simulink library "TTLibrary"  (R2015a)
settings: Solver=ode45  StartTime=0.0  StopTime=10.0  RelTol=1e-3
undefined symbols (not defined in the file): addNoise, aHeat, Area, b, cp, inputOpt, kl, Kv, L1i, p, sampleTime, T1i, tPause, uT1
settings Model: CovSFcnEnable=off  Creator=blindner  LastModifiedBy=blindner
settings DebuggingCC: SolverPrmCheckMsg=warning

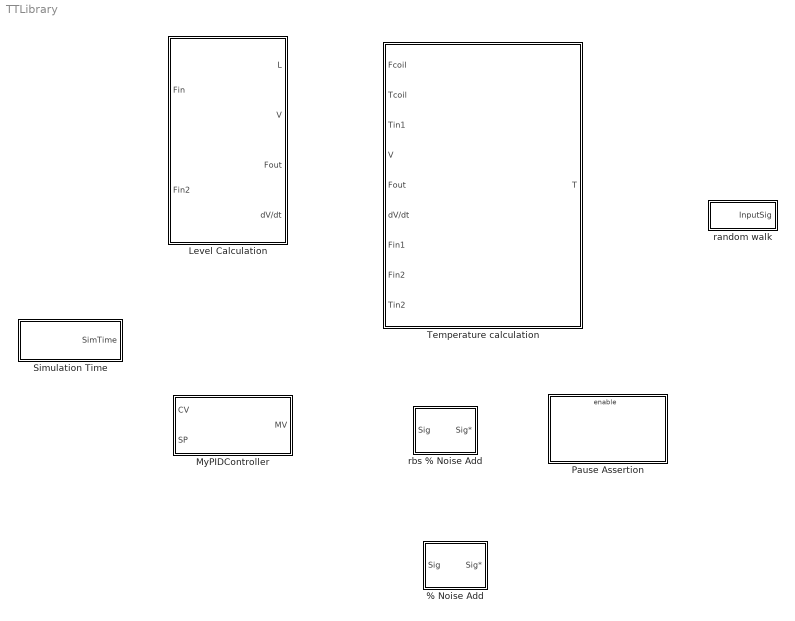
== system TTLibrary ==
  % Noise Add : Subsystem  mask{perc=5, seed=randi(100000), addNoiseMult=addNoise, Ts=sampleTime, noiseAmp=0}
      mask prompts: perc "Percentage Noise Added"; addNoiseMult "Add Noise: 0 or 1"; Ts "Sample Time"; noiseAmp "Amplitude of Noise added"
      mask Display: fprintf('AddNoise')
  Level Calculation : Subsystem  mask{kl=kl, Area=Area, Li=L1i, numIn=2}
      mask prompts: kl "Proportionality Constant"; Area "Cross-sectional Area"; Li "Initial Level"; numIn "Number of inports"
      mask init:
      | block = find_system(gcb,...
      |     'LookUnderMasks','on',...
      |     'FollowLinks','on','Name','Fin2');
      | 
      | switch numIn
      |     case '1'
      |         if ~isempty(block)
      |             delete_line(gcb,'Fin2/1','Sum/3');
      |             delete_block(block);
      |             set_param([gcb,'/Sum'],'Inputs','|+-')
      |         end
      |     case '2'
      |         if isempty(block)
      |             add_block('built-in/Inport',[gcb,'/Fin2'], 'Position',[155 190 175 210]);
      |            
      |             set_param([gcb,'/Sum'],'Inputs','+-+')
      |             add_line(gcb,'Fin2/1','Sum/3','autorouting','on');
      |             
      |         end
      | end % switch
      mask TypeOptions numIn: 1 | 2
  MyPIDController : Subsystem  mask{Kc=0, TI=0, Td=0, kv=0}
      mask prompts: Kc "Controller Gain"; TI "Integral Time"; Td "Derivative Time"; kv "Valve Constant"
      mask DialogControl DescTextVar Prompt: MV(s)=Kc*(1+1/TIs+Tds)*E(s)
  Pause Assertion : Subsystem
  Simulation Time : Subsystem  Variant=on  OverrideUsingVariant=Variant
  Temperature calculation : Subsystem  mask{Ti=T1i, p=p, cp=cp, b=b, aHeat=aHeat, numIn=2}
      mask prompts: Ti "Initial Temperature"; p "Density"; cp "Heat Capacity"; b "b: Heat transfer coeff costant"; aHeat "aHeat: Heat transfer coeff constant"; numIn "Number of Inports"
      mask init:
      | block = find_system(gcb,...
      |     'LookUnderMasks','on',...
      |     'FollowLinks','on','Name','Fin2');
      | 
      | switch numIn
      |     case '1'
      |         if ~isempty(block)
      |             delete_line(gcb,'Fin2/1','NewProduct/1');
      |             delete_line(gcb,'Tin2/1','NewProduct/2');
      |             delete_line(gcb,'NewProduct/1','Sum4/4');
      |             delete_block(block);
      |             delete_block([gcb,'/Tin2']);
      |             delete_block([gcb,'/NewProduct']);
      |             set_param([gcb,'/Sum4'],'Inputs','-+-')
      |           
      |         end
      |     case '2'
      |         if isempty(block)
      |             add_block('built-in/Inport',[gcb,'/Fin2'],'Position',[180   143   210   157]);
      |             add_block('built-in/Inport',[gcb,'/Tin2'],'Position',[180   173   210   187]);
      |             add_block('built-in/Product',[gcb,'/NewProduct'],'Position',[425   133   450   197]);
      |             
      |             set_param([gcb,'/Sum4'],'Inputs','-+-+')
      |             add_line(gcb,'Fin2/1','NewProduct/1','autorouting','on');
      |             add_line(gcb,'Tin2/1','NewProduct/2','autorouting','on');
      |             add_line(gcb,'NewProduct/1','Sum4/4','autorouting','on');
      |             
      |         end
      | end % switch
      mask TypeOptions numIn: 1 | 2
  random walk : Subsystem  mask{addNoise=0, noiseSeed=0, sampleTime=1, grad=0.1, IC=0, UB=1, LB=0}
      mask prompts: addNoise "Add Noise: 0 or 1"; noiseSeed "Seed for Random Number Generator"; sampleTime "Sample Time"; grad "Random walk slope"; IC "Initial condition"; UB "Upper bound for input"; LB "Lower bound for input"
      mask DialogControl DescTextVar Prompt: Simulates Random Walks on Inputs to Introduce Process Noise
  rbs % Noise Add : Subsystem  mask{perc=5, seed=randi(100000), u=uT1, addNoiseMult=addNoise}
      mask prompts: perc "Percentage Noise Added"; u "RBS input from workspace"; addNoiseMult "Add Noise: 0 or 1"

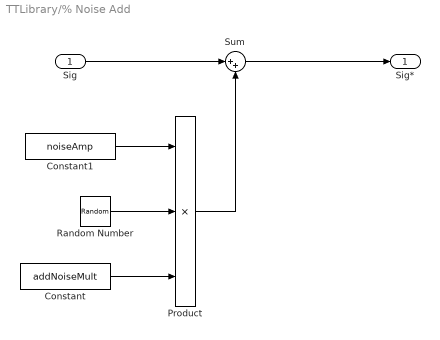
== system TTLibrary/% Noise Add ==
  Sig : Inport
  Constant : Constant  Value=addNoiseMult
  Constant1 : Constant  Value=noiseAmp
  Product : Product  Inputs=3
  Random Number : RandomNumber  Variance=perc/100  Seed=seed  SampleTime=Ts
  Sum : Sum  Inputs=|++
  Sig* : Outport
  wires:
  Sum/1 -> Sig*/1
  Product/1 -> Sum/2
  Sig/1 -> Sum/1
  Random Number/1 -> Product/2
  Constant/1 -> Product/3
  Constant1/1 -> Product/1

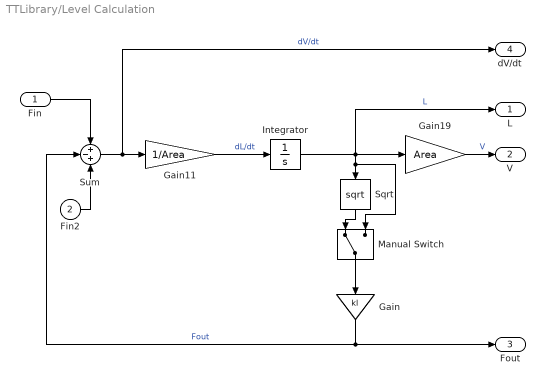
== system TTLibrary/Level Calculation ==
  Fin : Inport
  Fin2 : Inport  Port=2
  Gain : Gain  Gain=kl
  Gain11 : Gain  Gain=1/Area
  Gain19 : Gain  Gain=Area
  Integrator : Integrator  InitialCondition=Li
  Manual Switch : ManualSwitch
  Sqrt : Sqrt  SaturateOnIntegerOverflow=on
  Sum : Sum  Inputs=+-+
  L : Outport
  V : Outport  Port=2
  Fout : Outport  Port=3
  dV/dt : Outport  Port=4
  wires:
  Gain11/1 -> Integrator/1  "dL/dt"
  Integrator/1 -> Gain19/1, L/1, Manual Switch/2, Sqrt/1  "L"
  Fin/1 -> Sum/1
  Sum/1 -> dV/dt/1, Gain11/1  "dV/dt"
  Gain19/1 -> V/1  "V"
  Sqrt/1 -> Manual Switch/1
  Gain/1 -> Sum/2, Fout/1  "Fout"
  Fin2/1 -> Sum/3
  Manual Switch/1 -> Gain/1

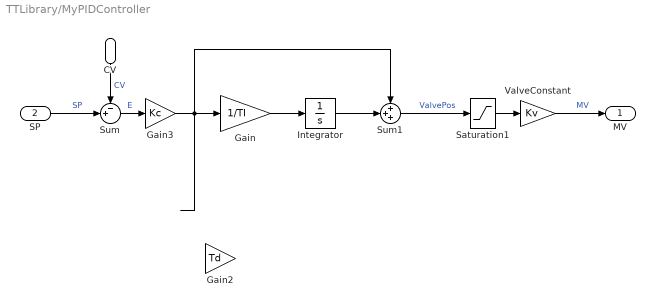
== system TTLibrary/MyPIDController ==
  CV : Inport
  SP : Inport  Port=2
  Gain : Gain  Gain=1/TI
  Gain2 : Gain  Gain=Td
  Gain3 : Gain  Gain=Kc
  Integrator : Integrator
  Saturation1 : Saturate  UpperLimit=inf  LowerLimit=0
  Sum : Sum  Inputs=-+|
  Sum1 : Sum  Inputs=+++
  ValveConstant : Gain  Gain=Kv
  MV : Outport
  wires:
  Sum1/1 -> Saturation1/1  "ValvePos"
  SP/1 -> Sum/2  "SP"
  Sum/1 -> Gain3/1  "E"
  CV/1 -> Sum/1  "CV"
  ValveConstant/1 -> MV/1  "MV"
  Saturation1/1 -> ValveConstant/1
  Gain3/1 -> Gain/1, Sum1/1
  Integrator/1 -> Sum1/2
  Gain/1 -> Integrator/1
  ? -> Sum1/3

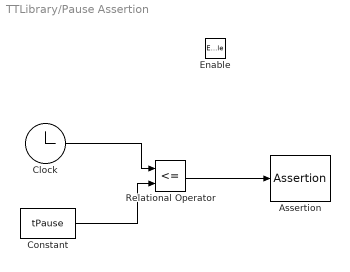
== system TTLibrary/Pause Assertion ==
  Enable : EnablePort
  Assertion : Assertion  AssertionFailFcn=set_param(bdroot,'SimulationCommand','pause')  StopWhenAssertionFail=off
  Clock : Clock
  Constant : Constant  Value=tPause
  Relational Operator : RelationalOperator  Operator=<=  OutDataTypeStr=boolean
  wires:
  Clock/1 -> Relational Operator/1
  Relational Operator/1 -> Assertion/1
  Constant/1 -> Relational Operator/2

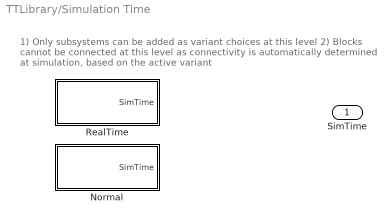
== system TTLibrary/Simulation Time ==
  note: 1) Only subsystems can be added as variant choices at this level
      | 2) Blocks cannot be connected at this level as connectivity is
      | automatically determined at simulation, based on the active variant
  Normal : Subsystem  VariantControl=Variant1
  RealTime : Subsystem  VariantControl=Variant
  SimTime : Outport

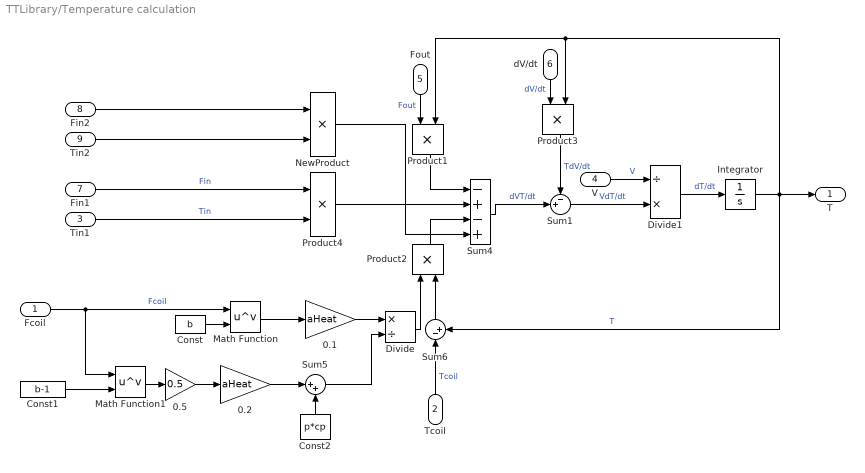
== system TTLibrary/Temperature calculation ==
  Fcoil : Inport
  Tcoil : Inport  Port=2
  Tin1 : Inport  Port=3
  V : Inport  Port=4
  Fout : Inport  Port=5
  dV/dt : Inport  Port=6
  Fin1 : Inport  Port=7
  Fin2 : Inport  Port=8
  Tin2 : Inport  Port=9
  0.1 : Gain  Gain=aHeat
  0.2 : Gain  Gain=aHeat
  0.5 : Gain  Gain=0.5
  Const : Constant  Value=b
  Const1 : Constant  Value=b-1
  Const2 : Constant  Value=p*cp
  Divide : Product  Inputs=*/
  Divide1 : Product  Inputs=/*
  Integrator : Integrator  InitialCondition=Ti
  Math Function : Math  Operator=pow  SaturateOnIntegerOverflow=on
  Math Function1 : Math  Operator=pow  SaturateOnIntegerOverflow=on
  NewProduct : Product  SaturateOnIntegerOverflow=on  RndMeth=Zero  InputSameDT=on  OutDataTypeStr=Inherit: Same as first input
  Product{1..4} (4 alike) : Product  RndMeth=Zero
  Sum1 : Sum  Inputs=-+|
  Sum4 : Sum  Inputs=-+-+
  Sum5 : Sum  Inputs=|++
  Sum6 : Sum  Inputs=|-+
  "T " : Outport
  wires:
  Const2/1 -> Sum5/2
  Product1/1 -> Sum4/1
  Sum6/1 -> Product2/2
  Sum5/1 -> Divide/2
  Math Function1/1 -> 0.5/1
  0.2/1 -> Sum5/1
  Divide/1 -> Product2/1
  Product2/1 -> Sum4/3
  Integrator/1 -> "T "/1, Product3/2, Product1/2, Sum6/2  "T"
  V/1 -> Divide1/1  "V"
  Const/1 -> Math Function/2
  Divide1/1 -> Integrator/1  "dT/dt"
  Math Function/1 -> 0.1/1
  Const1/1 -> Math Function1/2
  0.1/1 -> Divide/1
  dV/dt/1 -> Product3/1  "dV/dt"
  Sum1/1 -> Divide1/2  "VdT/dt"
  Product3/1 -> Sum1/1  "TdV/dt"
  Sum4/1 -> Sum1/2  "dVT/dt"
  Fout/1 -> Product1/1  "Fout"
  Fcoil/1 -> Math Function/1, Math Function1/1  "Fcoil"
  0.5/1 -> 0.2/1
  Tcoil/1 -> Sum6/1  "Tcoil"
  Product4/1 -> Sum4/2
  Fin1/1 -> Product4/1  "Fin"
  Tin1/1 -> Product4/2  "Tin"
  Fin2/1 -> NewProduct/1
  Tin2/1 -> NewProduct/2
  NewProduct/1 -> Sum4/4

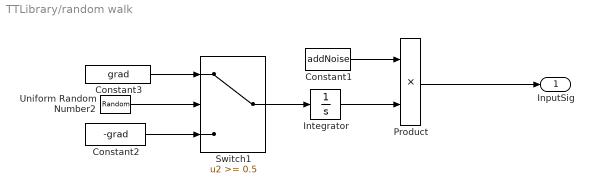
== system TTLibrary/random walk ==
  Constant1 : Constant  Value=addNoise
  Constant2 : Constant  Value=-grad
  Constant3 : Constant  Value=grad
  Integrator : Integrator  InitialCondition=IC  LimitOutput=on  UpperSaturationLimit=UB  LowerSaturationLimit=LB
  Product : Product
  Switch1 : Switch  Threshold=0.5
  Uniform Random Number2 : UniformRandomNumber  Minimum=0  Seed=noiseSeed  SampleTime=sampleTime
  InputSig : Outport
  wires:
  Product/1 -> InputSig/1
  Constant1/1 -> Product/1
  Constant3/1 -> Switch1/1
  Switch1/1 -> Integrator/1
  Constant2/1 -> Switch1/3
  Integrator/1 -> Product/2
  Uniform Random Number2/1 -> Switch1/2

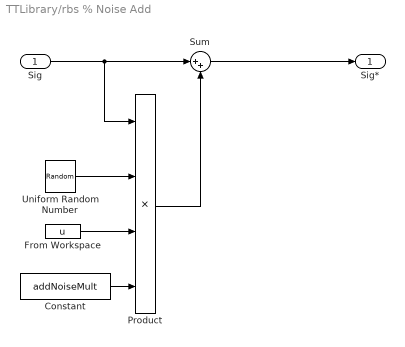
== system TTLibrary/rbs % Noise Add ==
  Sig : Inport
  Constant : Constant  Value=addNoiseMult
  From Workspace : FromWorkspace  VariableName=u  SampleTime=inputOpt.sampleTime  Interpolate=off  OutputAfterFinalValue=Cyclic repetition
  Product : Product  Inputs=4
  Sum : Sum  Inputs=|++
  Uniform Random Number : UniformRandomNumber  Minimum=-perc/100  Maximum=perc/100  Seed=seed  SampleTime=0.1
  Sig* : Outport
  wires:
  From Workspace/1 -> Product/3
  Sum/1 -> Sig*/1
  Product/1 -> Sum/2
  Sig/1 -> Sum/1, Product/1
  Uniform Random Number/1 -> Product/2
  Constant/1 -> Product/4

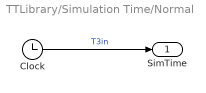
== system TTLibrary/Simulation Time/Normal ==
  Clock : Clock
  SimTime : Outport
  wires:
  Clock/1 -> SimTime/1  "T3in"

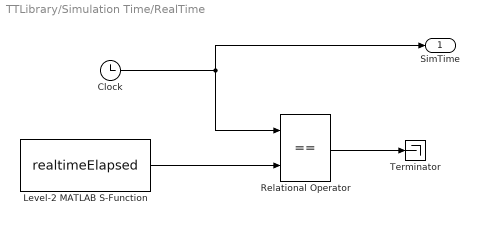
== system TTLibrary/Simulation Time/RealTime ==
  Clock : Clock
  Level-2 MATLAB S-Function : M-S-Function  FunctionName=realtimeElapsed
  Relational Operator : RelationalOperator  Operator===  OutDataTypeStr=boolean
  Terminator : Terminator
  SimTime : Outport
  wires:
  Level-2 MATLAB S-Function/1 -> Relational Operator/2
  Clock/1 -> Relational Operator/1, SimTime/1
  Relational Operator/1 -> Terminator/1
